simulink model "closedloop"  (R2017a)
settings: Solver=VariableStepAuto  StartTime=0.0  StopTime=Tf  MaxStep=1e-6  RelTol=1e-3
values from neighbouring files (symbols this model uses):
  den_Gpf = num_Go(end)    [Lab_7.m]
  num_Gpf = den_Go(end)    [Lab_7.m]
undefined symbols (not defined in the file or in its folder): den_Gc, den_Gp, num_Gc, num_Gp
settings Model: Creator=localmgr  LastModifiedBy=localmgr

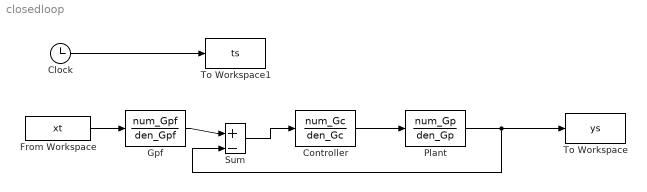
== system closedloop ==
  Clock : Clock
  Controller : TransferFcn  Numerator=num_Gc  Denominator=den_Gc
  From Workspace : FromWorkspace  VariableName=xt  SampleTime=0
  Gpf : TransferFcn  Numerator=num_Gpf  Denominator=den_Gpf
  Plant : TransferFcn  Numerator=num_Gp  Denominator=den_Gp
  Sum : Sum  Inputs=|+|||-|
  To Workspace : ToWorkspace  VariableName=ys  SampleTime=-1
  To Workspace1 : ToWorkspace  VariableName=ts  SampleTime=-1
  wires:
  Plant/1 -> Sum/2, To Workspace/1
  Clock/1 -> To Workspace1/1
  Controller/1 -> Plant/1
  Sum/1 -> Controller/1
  From Workspace/1 -> Gpf/1
  Gpf/1 -> Sum/1
